simulink model "tank_system"  (R2018b)
settings: Solver=VariableStepAuto  StartTime=0.0  StopTime=10.0  RelTol=1e-3
values from neighbouring files (symbols this model uses):
  hmax = 10    [main.m]
undefined symbols (not defined in the file or in its folder): h10, h20
settings Model: Creator=fredericovaz  LastModifiedBy=fredericovaz

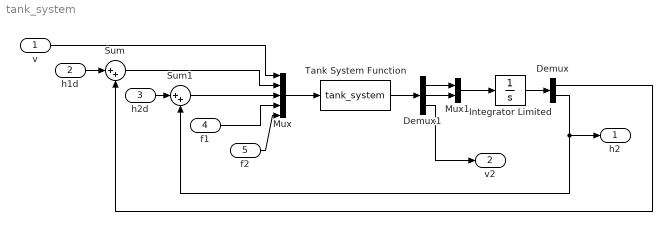
== system tank_system ==
  v : Inport
  h1d : Inport  Port=2
  h2d : Inport  Port=3
  f1 : Inport  Port=4
  f2 : Inport  Port=5
  Demux : Demux  Outputs=2
  Demux1 : Demux  Outputs=3
  Integrator Limited : Integrator  InitialCondition=[h10 h20]'  LimitOutput=on  UpperSaturationLimit=hmax  LowerSaturationLimit=0
  Mux : Mux  Inputs=5
  Mux1 : Mux  Inputs=2
  Sum : Sum  Inputs=|++
  Sum1 : Sum  Inputs=|++
  Tank System Function : MATLABFcn  MATLABFcn=tank_system  OutputDimensions=3
  h2 : Outport
  v2 : Outport  Port=2
  wires:
  Tank System Function/1 -> Demux1/1
  Mux/1 -> Tank System Function/1
  v/1 -> Mux/1
  f1/1 -> Mux/4
  f2/1 -> Mux/5
  Demux1/1 -> Mux1/1
  Demux1/2 -> Mux1/2
  Mux1/1 -> Integrator Limited/1
  Integrator Limited/1 -> Demux/1
  Demux1/3 -> v2/1
  Sum/1 -> Mux/2
  h1d/1 -> Sum/1
  Demux/1 -> Sum/2
  Demux/2 -> h2/1, Sum1/2
  h2d/1 -> Sum1/1
  Sum1/1 -> Mux/3
